simulink model "Lab_10"  (R2024b)
settings: Solver=VariableStepAuto  StartTime=0.0  StopTime=10.0  RelTol=1e-3
libraries: simulink x1, spsMonostableLib x1, spsSawtoothGeneratorLib x1
settings Model: LastModifiedBy=LENOVO

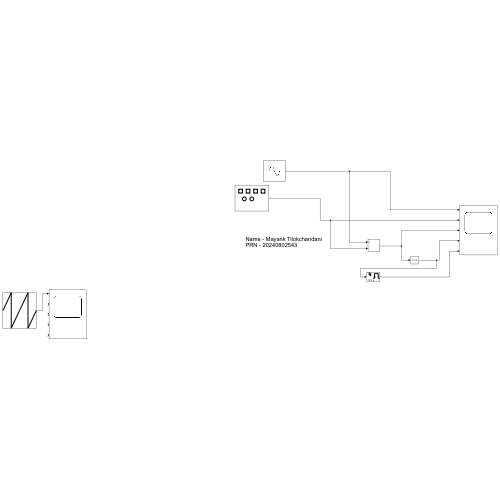
[thumbnail: Simulink's stored preview of the top-level diagram]
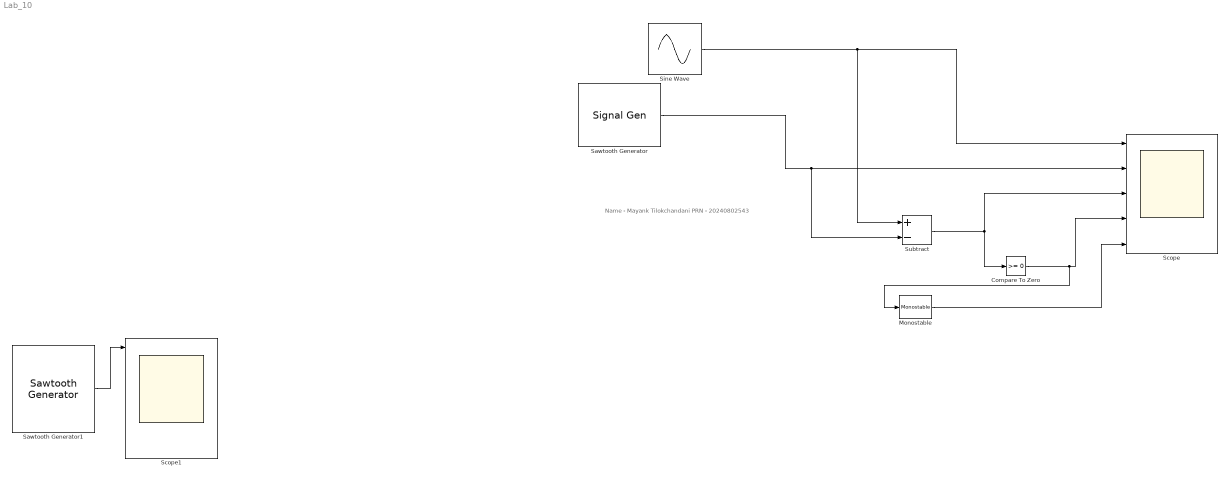
== system Lab_10 ==
  note: Name - Mayank Tilokchandani
      | PRN - 20240802543
  Compare To Zero : simulink/Logic and Bit Operations/Compare To Zero  relop=>=  OutDataTypeStr=boolean
  Monostable : spsMonostableLib/Monostable  EdgeDetect=Falling  PulseDuration=0.5  ic=0  Ts=0
      settings: LibrarySourceBlock=sps_lib/Control/Monostable
  Sawtooth Generator : SignalGenerator  WaveForm=sawtooth  Frequency=2*pi*1  Units=rad/sec
  Sawtooth Generator1 : spsSawtoothGeneratorLib/Sawtooth Generator  Freq=1e3  Phase=180  Ts=0
  Scope : Scope  NumInputPorts=5
  Scope1 : Scope  NumInputPorts=5
  Sine Wave : Sin  SampleTime=0
  Subtract : Sum  Inputs=+-
  wires:
  Sine Wave/1 -> Scope/1, Subtract/1
  Sawtooth Generator/1 -> Subtract/2, Scope/2
  Subtract/1 -> Compare To Zero/1, Scope/3
  Compare To Zero/1 -> Monostable/1, Scope/4
  Monostable/1 -> Scope/5
  Sawtooth Generator1/1 -> Scope1/1
